simulink model "adrc"  (R2022b)
settings: Solver=VariableStepAuto  StartTime=0.0  StopTime=30  RelTol=1e-3
model workspace (MAT data in the model file):
  HIGH = Simulink.Parameter
  HIGH.Value = 1
  HIGH.DataType = 'uint8'
  HIGH.Complexity = 'real'
  HIGH.Dimensions = [1 1]
  LOW = Simulink.Parameter
  LOW.Value = 0
  LOW.DataType = 'uint8'
  LOW.Complexity = 'real'
  LOW.Dimensions = [1 1]
settings Model: PacingRate=0.890000  Creator=wyq  LastModifiedBy=wyq

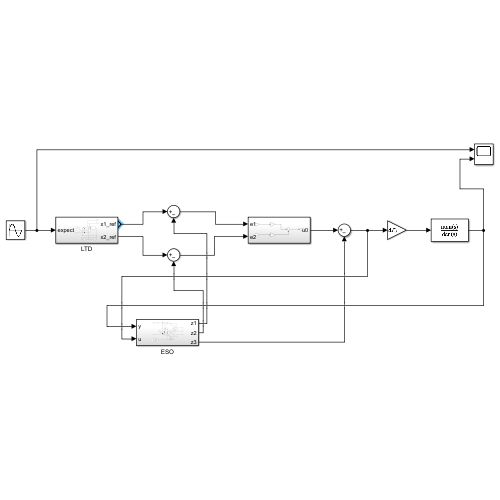
[thumbnail: Simulink's stored preview of the top-level diagram]
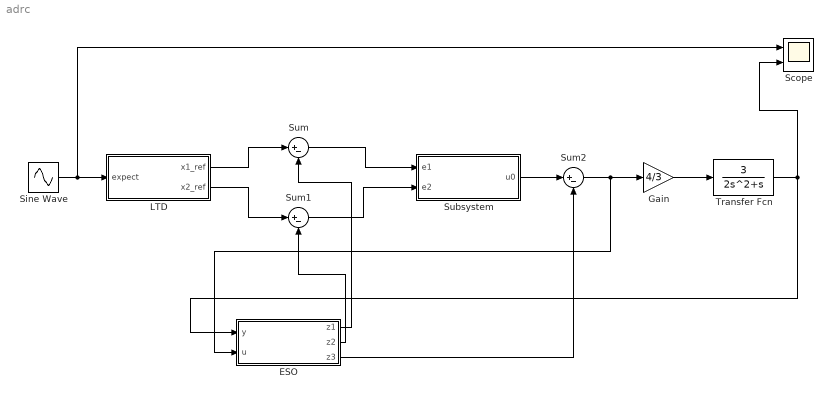
== system adrc ==
  ESO : Subsystem
  Gain : Gain  Gain=4/3
  LTD : Subsystem
  Scope : Scope  NumInputPorts=2
  Sine Wave : Sin  SampleTime=0
  Subsystem : Subsystem
  Sum : Sum  Inputs=|+-
  Sum1 : Sum  Inputs=|+-
  Sum2 : Sum  Inputs=|+-
  Transfer Fcn : TransferFcn  Numerator=[3]  Denominator=[2 1 0]
  wires:
  Sum1/1 -> Subsystem/2(e2)
  Sum/1 -> Subsystem/1(e1)
  LTD/1(x1_ref) -> Sum/1
  LTD/2(x2_ref) -> Sum1/1
  ESO/1(z1) -> Sum/2
  ESO/2(z2) -> Sum1/2
  ESO/3(z3) -> Sum2/2
  Subsystem/1(u0) -> Sum2/1
  Sum2/1 -> ESO/2(u), Gain/1
  Gain/1 -> Transfer Fcn/1
  Transfer Fcn/1 -> Scope/2, ESO/1(y)
  Sine Wave/1 -> Scope/1, LTD/1(expect)

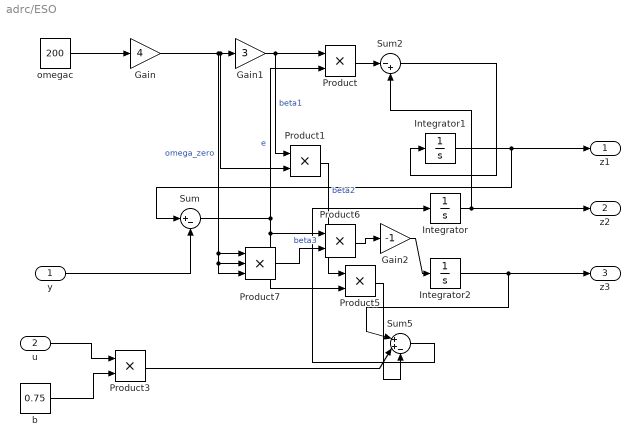
== system adrc/ESO ==
  y : Inport
  u : Inport  Port=2
  Gain : Gain  Gain=4
  Gain1 : Gain  Gain=3
  Gain2 : Gain  Gain=-1
  Integrator : Integrator
  Integrator1 : Integrator
  Integrator2 : Integrator
  Product{,1,3,5..6} (5 alike) : Product
  Product7 : Product  Inputs=3
  Sum : Sum  Inputs=|+-
  Sum2 : Sum  Inputs=|-+
  Sum5 : Sum  Inputs=|++-
  b : Constant  Value=0.75
  omegac : Constant  Value=200
  z1 : Outport
  z2 : Outport  Port=2
  z3 : Outport  Port=3
  wires:
  omegac/1 -> Gain/1
  y/1 -> Sum/2
  Integrator1/1 -> Sum/1, z1/1
  Gain1/1 -> Product/1, Product1/1  "beta1"
  Sum/1 -> Product/2, Product6/1, Product5/2  "e"
  Gain/1 -> Product7/1, Product7/3, Product7/2, Product1/2, Gain1/1  "omega_zero"
  Sum2/1 -> Integrator1/1
  Integrator/1 -> z2/1, Sum2/2
  Integrator2/1 -> Sum5/1, z3/1
  Product7/1 -> Product6/2  "beta3"
  u/1 -> Product3/1
  b/1 -> Product3/2
  Product3/1 -> Sum5/2
  Product1/1 -> Product5/1  "beta2"
  Product5/1 -> Sum5/3
  Sum5/1 -> Integrator/1
  Product/1 -> Sum2/1
  Product6/1 -> Gain2/1
  Gain2/1 -> Integrator2/1

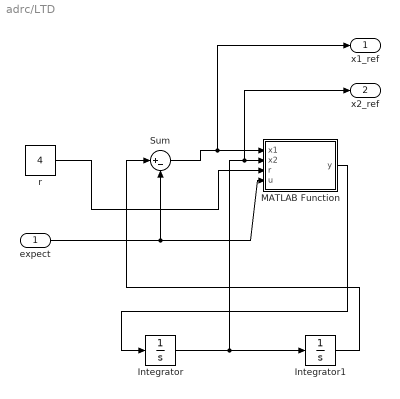
== system adrc/LTD ==
  expect : Inport
  Integrator : Integrator
  Integrator1 : Integrator
  MATLAB Function : MATLAB Function  TreatAsAtomicUnit=on
  Sum : Sum  Inputs=|+-
  r : Constant  Value=4
  x1_ref : Outport
  x2_ref : Outport  Port=2
  wires:
  MATLAB Function/1(y) -> Integrator/1
  r/1 -> MATLAB Function/3(r)
  Integrator/1 -> x2_ref/1, MATLAB Function/2(x2), Integrator1/1
  expect/1 -> Sum/2, MATLAB Function/4(u)
  Sum/1 -> x1_ref/1, MATLAB Function/1(x1)
  Integrator1/1 -> Sum/1

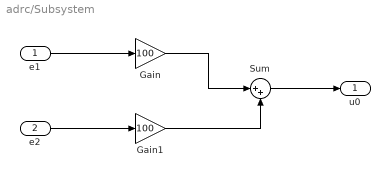
== system adrc/Subsystem ==
  e1 : Inport
  e2 : Inport  Port=2
  Gain : Gain  Gain=100
  Gain1 : Gain  Gain=100
  Sum : Sum  Inputs=|++
  u0 : Outport
  wires:
  e2/1 -> Gain1/1
  e1/1 -> Gain/1
  Sum/1 -> u0/1
  Gain1/1 -> Sum/2
  Gain/1 -> Sum/1

== matlab function adrc/LTD/MATLAB Function ==
  data: x1 input; x2 input; r input; u input; y output
function y = fcn(x1, x2, r, u)

y = -r*r*x1-2*r*x2+r*r*u;
